simulink model "Transmitter1"  (R2019b)
settings: Solver=FixedStepDiscrete  StartTime=0.0  StopTime=inf  FixedStep=0.02  RelTol=1e-3  EnableMultiTasking=on
undefined symbols (not defined in the file): Busy, Wait
libraries: aerolibanimutils x2, dspnetwork x1
settings Model: Creator=Jorg Angelov  LastModifiedBy=bhisma
settings DataIOCC: LimitDataPoints=on  SaveFormat=Array  ReturnWorkspaceOutputs=off
settings OptimizationCC: LifeSpan=inf
settings DebuggingCC: SolverPrmCheckMsg=warning  AllowSymbolicDim=off  SFUnexpectedBacktrackingDiag=warning  SFNoUnconditionalDefaultTransitionDiag=warning  ArithmeticOperatorsInVariantConditions=warning
settings HardwareCC: ProdBitPerPointer=32  ProdBitPerSizeT=32  ProdBitPerPtrDiffT=32  ProdLargestAtomicFloat=None  ProdIntDivRoundTo=Undefined  ProdEndianess=Unspecified  ProdWordSize=32  ProdHWDeviceType=32-bit Generic
settings ModelReferenceCC: PropagateSignalLabelsOutOfModel=off
settings SFSimCC: SimUseLocalCustomCode=off  CustomCodeUndefinedFunction=UseInterfaceOnly
settings RTWCC: RTWUseLocalCustomCode=off
settings CodeAppCC: StateflowObjectComments=on
settings GRTTargetCC: TargetLangStandard=C89/C90 (ANSI)  GeneratePreprocessorConditionals=Disable all
settings ConfigComp: CovMetricSettings=dw  CovHtmlReporting=on  CovSaveCumulativeToWorkspaceVar=on  CovSaveSingleToWorkspaceVar=on  CovExternalEMLEnable=off  CovSFcnEnable=off

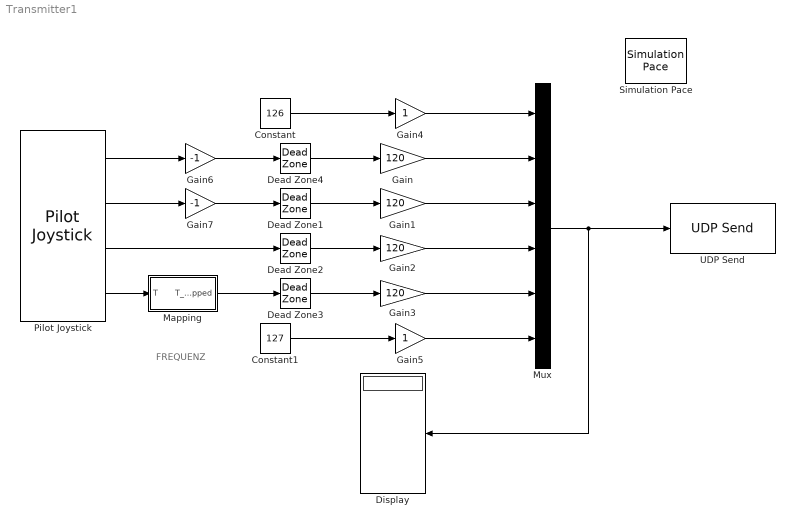
== system Transmitter1 ==
  note: FREQUENZ
  Constant : Constant  Value=126  OutDataTypeStr=int8
  Constant1 : Constant  Value=127  OutDataTypeStr=int8
  Dead Zone1 : DeadZone  LowerValue=-0.15  UpperValue=0.15  SaturateOnIntegerOverflow=on
  Dead Zone2 : DeadZone  LowerValue=-0.15  UpperValue=0.15  SaturateOnIntegerOverflow=on
  Dead Zone3 : DeadZone  LowerValue=-0.1  UpperValue=0.1  SaturateOnIntegerOverflow=on
  Dead Zone4 : DeadZone  LowerValue=-0.15  UpperValue=0.15  SaturateOnIntegerOverflow=on
  Display : Display
  Gain{,1..3} (4 alike) : Gain  Gain=120  OutDataTypeStr=int8
  Gain4 : Gain  OutDataTypeStr=int8
  Gain5 : Gain  OutDataTypeStr=int8
  Gain6 : Gain  Gain=-1  OutDataTypeStr=double
  Gain7 : Gain  Gain=-1  OutDataTypeStr=double
  Mapping : Subsystem  TreatAsAtomicUnit=on
  Mux : Mux  Inputs=6
  Pilot Joystick : aerolibanimutils/Pilot Joystick  JoystickID=Joystick1  OutputConfiguration=FourAxis  SampleTime=-1
  Simulation Pace : aerolibanimutils/Simulation Pace  SimulationPace=1  SleepMode=Busy-Wait  OutputPaceError=off  SampleTime=-1
  UDP Send : dspnetwork/UDP Send  remoteURL='255.255.255.255'  remotePort=1337  localURL='0.0.0.0'  localPortSource=Automatically determine  localPort=-1  sampletime=-1  blockPlatform=[]  separateLengthPort=0
      settings: SourceProductName=Simulink
  wires:
  Constant1/1 -> Gain5/1
  Mux/1 -> UDP Send/1, Display/1
  Constant/1 -> Gain4/1
  Gain/1 -> Mux/2
  Gain1/1 -> Mux/3
  Gain2/1 -> Mux/4
  Gain3/1 -> Mux/5
  Pilot Joystick/1 -> Gain6/1
  Pilot Joystick/2 -> Gain7/1
  Pilot Joystick/3 -> Dead Zone2/1
  Pilot Joystick/4 -> Mapping/1(T)
  Gain5/1 -> Mux/6
  Gain4/1 -> Mux/1
  Mapping/1(T_mapped) -> Dead Zone3/1
  Dead Zone4/1 -> Gain/1
  Dead Zone1/1 -> Gain1/1
  Dead Zone2/1 -> Gain2/1
  Dead Zone3/1 -> Gain3/1
  Gain6/1 -> Dead Zone4/1
  Gain7/1 -> Dead Zone1/1

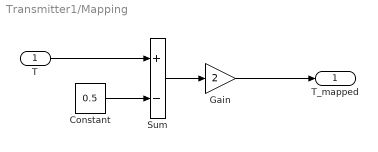
== system Transmitter1/Mapping ==
  T : Inport
  Constant : Constant  Value=0.5
  Gain : Gain  Gain=2
  Sum : Sum  Inputs=+-
  T_mapped : Outport
  wires:
  T/1 -> Sum/1
  Constant/1 -> Sum/2
  Sum/1 -> Gain/1
  Gain/1 -> T_mapped/1
